simulink model "gm_whdlOFDMTx"  (R2022b)
settings: Solver=FixedStepDiscrete  StartTime=0.0  StopTime=0  RelTol=1e-3
model workspace (MATLAB code in the model file):
  | config = whdlexamples.OFDMTxParameters();
  | fftLen = config.fftLen;
  | subC = config.subC;
  | cpLen = config.cpLen;
  | fs = config.fs;
  | NSS = config.NSS;
  | NRS = config.NRS;
  | NHeader = config.NHeader;
  | NData = config.NData;
  | NSymPerF = config.NSymPerF;
  | ssSymbol = config.ssSymbol;
  | rsSymbol = config.rsSymbol;
  | NHeaderBits = config.NHeaderBits;
  | headerCRCBool = config.headerCRCBool;
  | headerConvK = config.headerConvK;
  | headerConvCode = config.headerConvCode;
  | pilotValPerSym = config.pilotValPerSym;
  | pilotLen = config.pilotLen;
  | dataCRCPoly = config.dataCRCPoly;
  | dataCRCBool = config.dataCRCBool;
  | dataCRCLen = config.dataCRCLen;
  | dataConvK = config.dataConvK;
  | dataConvCode = config.dataConvCode;
  | scramInit = config.scramInit;
  | firCoeff = config.firCoeff;
  | rateFac1 = config.rateFac1;
  | rateFac2 = config.rateFac2;
  | headerLat = config.headerLat;
  | headerTime = config.headerTime;
  | preambleInd = config.preambleInd;
  | headerDataInd = config.headerDataInd;
  | trBlkSize = config.trBlkSize;
  | randOFDM = config.randOFDM;
  | headerIntrlvMaxBlkSize = config.headerIntrlvMaxBlkSize;
  | headerIntrlvNColumns   = config.headerIntrlvNColumns;
  | dataIntrlvMaxBlkSize   = config.dataIntrlvMaxBlkSize;
  | dataIntrlvNColumns     = config.dataIntrlvNColumns;
  | clear config
libraries: hdlsllib x49, simulink x22, dspsigops x11, whdlmod x3, whdledac x3, whdlutilities x2, commhdlcrc x2, dsphdlfiltering2 x1
(part 1 of 4)
settings Model: DataDictionary=whdlOFDMTxData.sldd  Creator=The MathWorks, Inc.  LastModifiedBy=Marwan
settings SolverCC: AlgebraicLoopSolver=TrustRegion  MaxZcPerStep=1
settings DataIOCC: VisualizeSimOutput=off  SaveTime=off  ReturnWorkspaceOutputs=off
settings OptimizationCC: BlockReduction=off  ConditionallyExecuteInputs=off  DefaultParameterBehavior=Inlined  InitFltsAndDblsToZero=on  EfficientMapNaN2IntZero=off
settings DebuggingCC: StringTruncationChecking=none  AlgebraicLoopMsg=error  InheritedTsInSrcMsg=none  SingleTaskRateTransMsg=error  UnconnectedInputMsg=warning  UnconnectedOutputMsg=warning  UnconnectedLineMsg=warning  SFMachineParentedDataDiag=warning
settings HardwareCC: ProdBitPerPointer=32  ProdBitPerSizeT=32  ProdBitPerPtrDiffT=32  ProdLargestAtomicFloat=None  ProdIntDivRoundTo=Undefined  ProdEndianess=Unspecified  ProdWordSize=32  ProdHWDeviceType=ASIC/FPGA->ASIC/FPGA  TargetBitPerPointer=64  TargetBitPerSizeT=64  TargetBitPerPtrDiffT=64  TargetLongLongMode=on  TargetIntDivRoundTo=Zero  TargetEndianess=LittleEndian  TargetWordSize=64  TargetHWDeviceType=Custom Processor->MATLAB Host Computer  ProdEqTarget=off
settings ModelReferenceCC: UpdateModelReferenceTargets=IfOutOfDate  EnableRefExpFcnMdlSchedulingChecks=on  ModelReferenceNumInstancesAllowed=Single
settings RTWCC: RTWVerbose=off  DLArmComputeVersion=19.05
settings CodeAppCC: GenerateComments=off  MaxIdLength=128

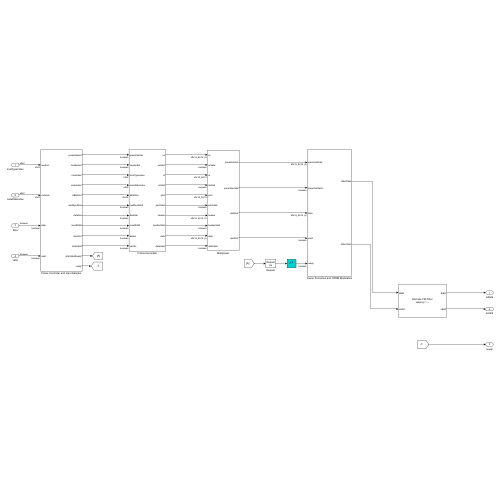
[thumbnail: Simulink's stored preview of the top-level diagram]
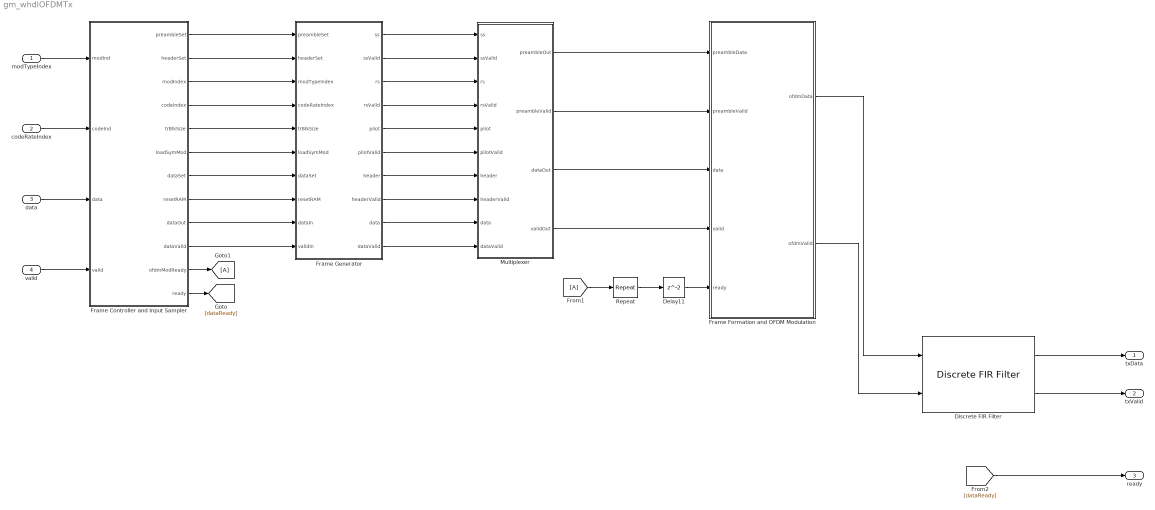
== system gm_whdlOFDMTx ==
  modTypeIndex : Inport  OutDataTypeStr=fixdt(0, 2, 0)  PortDimensions=1  SampleTime=4.8828125e-07
  codeRateIndex : Inport  Port=2  OutDataTypeStr=fixdt(0, 2, 0)  PortDimensions=1  SampleTime=4.8828125e-07
  data : Inport  Port=3  OutDataTypeStr=boolean  PortDimensions=1  SampleTime=4.8828125e-07
  valid : Inport  Port=4  OutDataTypeStr=boolean  PortDimensions=1  SampleTime=4.8828125e-07
  Delay11 : Delay
  Discrete FIR Filter : dsphdlfiltering2/Discrete FIR Filter  NumeratorSource=Property  Numerator=firCoeff  NumeratorPrototype=[]  FilterStructure=Direct form systolic  SerializationOption=Minimum number of cycles between valid input samples  NumCycles=2  NumberOfMultipliers=2  SimulateUsing=Code generation  roundingMode=Floor  overflowMode=off  CoefficientsDataTypeStr=Inherit: Same word length as input  OutputDataTypeStr=Inherit: Same word length as input  ResetInputPort=off  HDLGlobalReset=off
  Frame Controller and Input Sampler : Subsystem
  Frame Formation and OFDM Modulation : Subsystem
  Frame Generator : Subsystem
  From1 : From
  Goto1 : Goto
  Multiplexer : Subsystem
  Repeat : dspsigops/Repeat  N=2  RateOptions=Allow multirate processing  ic=0  mode=Unused parameter value
  txData : Outport  SampleTime=7.8125e-06  VectorParamsAs1DForOutWhenUnconnected=off
  txValid : Outport  Port=2  SampleTime=7.8125e-06  VectorParamsAs1DForOutWhenUnconnected=off
  ready : Outport  Port=3  SampleTime=4.8828125e-07  VectorParamsAs1DForOutWhenUnconnected=off
  wires:
  modTypeIndex/1 -> Frame Controller and Input Sampler/1(modInd)
  codeRateIndex/1 -> Frame Controller and Input Sampler/2(codeInd)
  data/1 -> Frame Controller and Input Sampler/3(data)
  valid/1 -> Frame Controller and Input Sampler/4(valid)
  Delay11/1 -> Frame Formation and OFDM Modulation/5(ready)
  Discrete FIR Filter/1 -> txData/1
  Discrete FIR Filter/2 -> txValid/1
  Frame Controller and Input Sampler/1(preambleSet) -> Frame Generator/1(preambleSet)
  Frame Controller and Input Sampler/2(headerSet) -> Frame Generator/2(headerSet)
  Frame Controller and Input Sampler/3(modIndex) -> Frame Generator/3(modTypeIndex)
  Frame Controller and Input Sampler/4(codeIndex) -> Frame Generator/4(codeRateIndex)
  Frame Controller and Input Sampler/5(trBlkSize) -> Frame Generator/5(trBlkSize)
  Frame Controller and Input Sampler/6(loadSymMod) -> Frame Generator/6(loadSymMod)
  Frame Controller and Input Sampler/7(dataSet) -> Frame Generator/7(dataSet)
  Frame Controller and Input Sampler/8(resetRAM) -> Frame Generator/8(resetRAM)
  Frame Controller and Input Sampler/9(dataOut) -> Frame Generator/9(dataIn)
  Frame Controller and Input Sampler/10(dataValid) -> Frame Generator/10(validIn)
  Frame Controller and Input Sampler/11(ofdmModReady) -> Goto1/1
  Frame Controller and Input Sampler/12(ready) -> [dataReady]
  Frame Formation and OFDM Modulation/1(ofdmData) -> Discrete FIR Filter/1
  Frame Formation and OFDM Modulation/2(ofdmValid) -> Discrete FIR Filter/2
  Frame Generator/1(ss) -> Multiplexer/1(ss)
  Frame Generator/2(ssValid) -> Multiplexer/2(ssValid)
  Frame Generator/3(rs) -> Multiplexer/3(rs)
  Frame Generator/4(rsValid) -> Multiplexer/4(rsValid)
  Frame Generator/5(pilot) -> Multiplexer/5(pilot)
  Frame Generator/6(pilotValid) -> Multiplexer/6(pilotValid)
  Frame Generator/7(header) -> Multiplexer/7(header)
  Frame Generator/8(headerValid) -> Multiplexer/8(headerValid)
  Frame Generator/9(data) -> Multiplexer/9(data)
  Frame Generator/10(dataValid) -> Multiplexer/10(dataValid)
  From1/1 -> Repeat/1
  [dataReady] -> ready/1
  Multiplexer/1(preambleOut) -> Frame Formation and OFDM Modulation/1(preambleData)
  Multiplexer/2(preambleValid) -> Frame Formation and OFDM Modulation/2(preambleValid)
  Multiplexer/3(dataOut) -> Frame Formation and OFDM Modulation/3(data)
  Multiplexer/4(validOut) -> Frame Formation and OFDM Modulation/4(valid)
  Repeat/1 -> Delay11/1

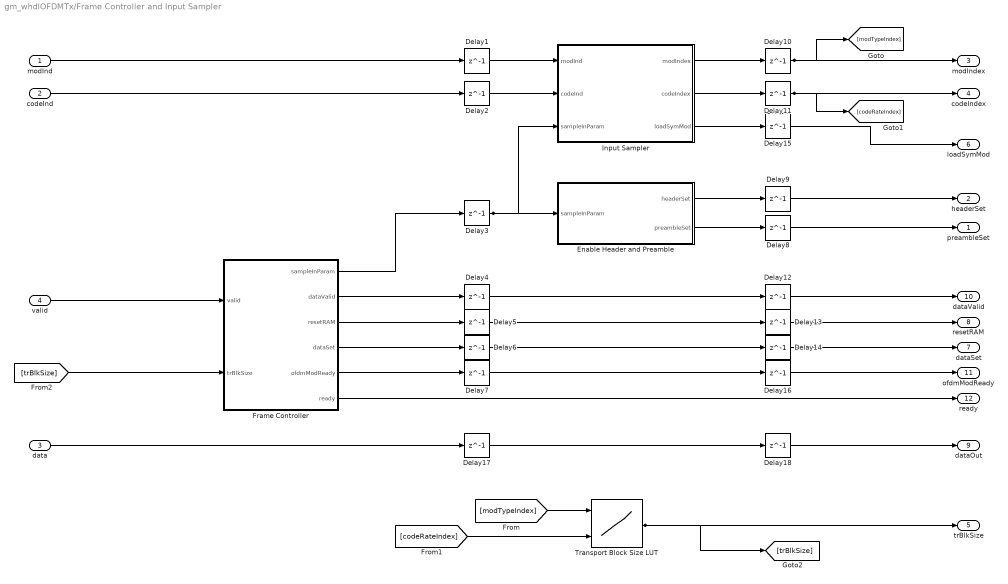
== system gm_whdlOFDMTx/Frame Controller and Input Sampler ==
  modInd : Inport  OutDataTypeStr=fixdt(0, 2, 0)  PortDimensions=1  SampleTime=4.8828125e-07
  codeInd : Inport  Port=2  OutDataTypeStr=fixdt(0, 2, 0)  PortDimensions=1  SampleTime=4.8828125e-07
  data : Inport  Port=3  OutDataTypeStr=boolean  PortDimensions=1  SampleTime=4.8828125e-07
  valid : Inport  Port=4  OutDataTypeStr=boolean  PortDimensions=1  SampleTime=4.8828125e-07
  Delay{1..18} (18 alike) : Delay  DelayLength=1
  "Enable Header and Preamble " : Subsystem
  Frame Controller : Subsystem
  Input Sampler : Subsystem
  Transport Block Size LUT : Lookup_n-D  BreakpointsForDimension1=0:3  BreakpointsForDimension2=0:3  IndexSearchMethod=Evenly spaced points  Table=trBlkSize  ExtrapMethod=Clip  DiagnosticForOutOfRangeInput=Error  UseLastTableValue=on  InternalRulePriority=Speed  OutDataTypeStr=fixdt(0,nextpow2(max(max(trBlkSize)) +1),0)  RndMeth=Simplest
      settings: InputPortMap=u0,u1
  preambleSet : Outport  SampleTime=4.8828125e-07
  headerSet : Outport  Port=2  SampleTime=4.8828125e-07
  modIndex : Outport  Port=3  SampleTime=4.8828125e-07
  codeIndex : Outport  Port=4  SampleTime=4.8828125e-07
  trBlkSize : Outport  Port=5  SampleTime=4.8828125e-07
  loadSymMod : Outport  Port=6  SampleTime=4.8828125e-07
  dataSet : Outport  Port=7  SampleTime=4.8828125e-07
  resetRAM : Outport  Port=8  SampleTime=4.8828125e-07
  dataOut : Outport  Port=9  SampleTime=4.8828125e-07
  dataValid : Outport  Port=10  SampleTime=4.8828125e-07
  ofdmModReady : Outport  Port=11  SampleTime=4.8828125e-07
  ready : Outport  Port=12  SampleTime=4.8828125e-07
  wires:
  modInd/1 -> Delay1/1
  codeInd/1 -> Delay2/1
  data/1 -> Delay17/1
  valid/1 -> Frame Controller/1(valid)
  Delay1/1 -> Input Sampler/1(modInd)
  Delay10/1 -> [modTypeIndex], modIndex/1
  Delay11/1 -> [codeRateIndex], codeIndex/1
  Delay12/1 -> dataValid/1
  Delay13/1 -> resetRAM/1
  Delay14/1 -> dataSet/1
  Delay15/1 -> loadSymMod/1
  Delay16/1 -> ofdmModReady/1
  Delay17/1 -> Delay18/1
  Delay18/1 -> dataOut/1
  Delay2/1 -> Input Sampler/2(codeInd)
  Delay3/1 -> Input Sampler/3(sampleInParam), "Enable Header and Preamble "/1(sampleInParam)
  Delay4/1 -> Delay12/1
  Delay5/1 -> Delay13/1
  Delay6/1 -> Delay14/1
  Delay7/1 -> Delay16/1
  Delay8/1 -> preambleSet/1
  Delay9/1 -> headerSet/1
  "Enable Header and Preamble "/1(headerSet) -> Delay9/1
  "Enable Header and Preamble "/2(preambleSet) -> Delay8/1
  Frame Controller/1(sampleInParam) -> Delay3/1
  Frame Controller/2(dataValid) -> Delay4/1
  Frame Controller/3(resetRAM) -> Delay5/1
  Frame Controller/4(dataSet) -> Delay6/1
  Frame Controller/5(ofdmModReady) -> Delay7/1
  Frame Controller/6(ready) -> ready/1
  [modTypeIndex] -> Transport Block Size LUT/1
  [codeRateIndex] -> Transport Block Size LUT/2
  [trBlkSize] -> Frame Controller/2(trBlkSize)
  Input Sampler/1(modIndex) -> Delay10/1
  Input Sampler/2(codeIndex) -> Delay11/1
  Input Sampler/3(loadSymMod) -> Delay15/1
  Transport Block Size LUT/1 -> [trBlkSize], trBlkSize/1

== system gm_whdlOFDMTx/Frame Formation and OFDM Modulation ==
  preambleData : Inport  OutDataTypeStr=fixdt(1, 16, 14)  PortDimensions=1  SampleTime=2.44140625e-07
      settings: SignalType=complex
  preambleValid : Inport  Port=2  OutDataTypeStr=boolean  PortDimensions=1  SampleTime=2.44140625e-07
  data : Inport  Port=3  OutDataTypeStr=fixdt(1, 16, 14)  PortDimensions=1  SampleTime=2.44140625e-07
      settings: SignalType=complex
  valid : Inport  Port=4  OutDataTypeStr=boolean  PortDimensions=1  SampleTime=2.44140625e-07
  ready : Inport  Port=5  OutDataTypeStr=boolean  PortDimensions=1  SampleTime=2.44140625e-07
  Complex to Real-Imag : ComplexToRealImag  Output=Real
  Data Type Conversion : DataTypeConversion  SaturateOnIntegerOverflow=off  RndMeth=Floor
  Delay3 : Delay  DelayLength=1
  Downsample : DownSample  N=rateFac1  RateOptions=Allow multirate processing
  Dual Rate RAM : hdlsllib/HDL RAMs/Dual Rate Dual Port RAM  ram_size=nextpow2(subC*NSymPerF +1)
  Dual Rate RAM_term0 : Terminator
  Generate OFDM Modulator Valid : Subsystem
  Generate RAM Inputs : Subsystem
  Make OFDM Valid Continuous : Subsystem
  OFDM Modulator : Subsystem
  constant : Constant  Value=complex(0)  OutDataTypeStr=Inherit: Inherit via back propagation  SampleTime=-1
  ofdmData : Outport  SampleTime=7.8125e-06  VectorParamsAs1DForOutWhenUnconnected=off
  ofdmValid : Outport  Port=2  SampleTime=7.8125e-06  VectorParamsAs1DForOutWhenUnconnected=off
  wires:
  preambleData/1 -> Generate RAM Inputs/1(preambleData)
  preambleValid/1 -> Generate RAM Inputs/2(enb)
  data/1 -> Generate RAM Inputs/3(data)
  valid/1 -> Generate RAM Inputs/4(valid)
  ready/1 -> Downsample/1
  Complex to Real-Imag/1 -> Data Type Conversion/1
  Data Type Conversion/1 -> Dual Rate RAM/6
  Delay3/1 -> Generate OFDM Modulator Valid/2(ofdmModReady)
  Downsample/1 -> Generate OFDM Modulator Valid/1(generatedReady)
  Dual Rate RAM/1 -> Dual Rate RAM_term0/1
  Dual Rate RAM/2 -> OFDM Modulator/1(data)
  Generate OFDM Modulator Valid/1(RAMAddress) -> Dual Rate RAM/5
  Generate OFDM Modulator Valid/2(ofdmModValid) -> OFDM Modulator/2(valid)
  Generate RAM Inputs/1(RAMData) -> Dual Rate RAM/1
  Generate RAM Inputs/2(RAMAddress) -> Dual Rate RAM/2
  Generate RAM Inputs/3(RAMValid) -> Dual Rate RAM/3
  Make OFDM Valid Continuous/1(ofdmData) -> ofdmData/1
  Make OFDM Valid Continuous/2(ofdmValid) -> ofdmValid/1
  OFDM Modulator/1(data1) -> Make OFDM Valid Continuous/1(dataIn)
  OFDM Modulator/2(valid1) -> Make OFDM Valid Continuous/2(validIn)
  OFDM Modulator/3(ready) -> Delay3/1
  constant/1 -> Complex to Real-Imag/1, Dual Rate RAM/4

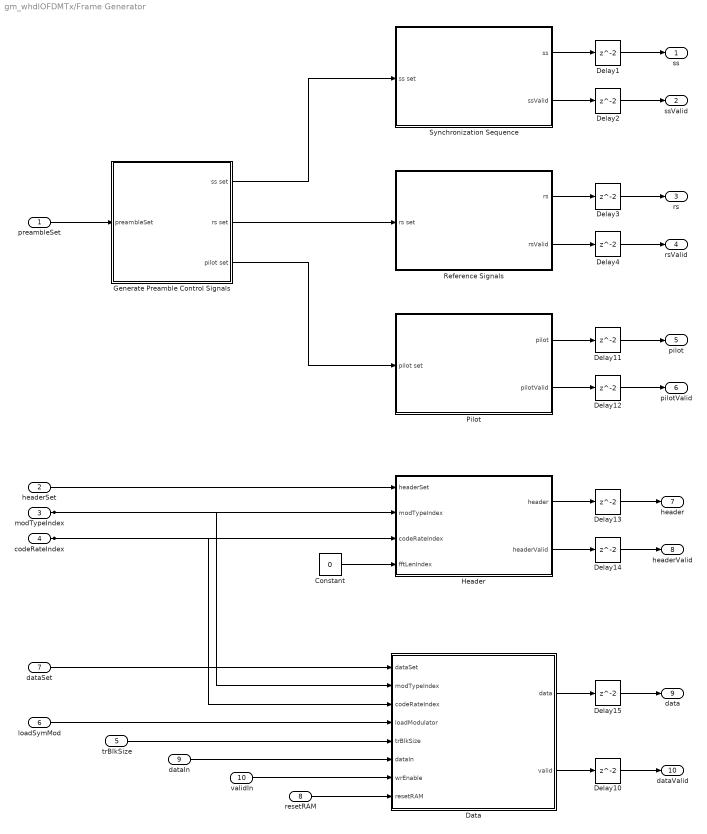
== system gm_whdlOFDMTx/Frame Generator ==
  preambleSet : Inport  OutDataTypeStr=boolean  PortDimensions=1  SampleTime=4.8828125e-07
  headerSet : Inport  Port=2  OutDataTypeStr=boolean  PortDimensions=1  SampleTime=4.8828125e-07
  modTypeIndex : Inport  Port=3  OutDataTypeStr=fixdt(0, 2, 0)  PortDimensions=1  SampleTime=4.8828125e-07
  codeRateIndex : Inport  Port=4  OutDataTypeStr=fixdt(0, 2, 0)  PortDimensions=1  SampleTime=4.8828125e-07
  trBlkSize : Inport  Port=5  OutDataTypeStr=fixdt(0, 14, 0)  PortDimensions=1  SampleTime=4.8828125e-07
  loadSymMod : Inport  Port=6  OutDataTypeStr=boolean  PortDimensions=1  SampleTime=4.8828125e-07
  dataSet : Inport  Port=7  OutDataTypeStr=boolean  PortDimensions=1  SampleTime=4.8828125e-07
  resetRAM : Inport  Port=8  OutDataTypeStr=boolean  PortDimensions=1  SampleTime=4.8828125e-07
  dataIn : Inport  Port=9  OutDataTypeStr=boolean  PortDimensions=1  SampleTime=4.8828125e-07
  validIn : Inport  Port=10  OutDataTypeStr=boolean  PortDimensions=1  SampleTime=4.8828125e-07
  Constant : Constant  Value=0  OutDataTypeStr=fixdt(0,3,0)  SampleTime=-1
  Data : Subsystem
  Delay{1..4,10..15} (10 alike) : Delay
  Generate Preamble Control Signals : Subsystem
  Header : Subsystem
  Pilot : Subsystem
  Reference Signals : Subsystem
  Synchronization Sequence : Subsystem
  ss : Outport  SampleTime=2.44140625e-07
  ssValid : Outport  Port=2  SampleTime=2.44140625e-07
  rs : Outport  Port=3  SampleTime=2.44140625e-07
  rsValid : Outport  Port=4  SampleTime=2.44140625e-07
  pilot : Outport  Port=5  SampleTime=2.44140625e-07
  pilotValid : Outport  Port=6  SampleTime=2.44140625e-07
  header : Outport  Port=7  SampleTime=2.44140625e-07
  headerValid : Outport  Port=8  SampleTime=2.44140625e-07
  data : Outport  Port=9  SampleTime=2.44140625e-07
  dataValid : Outport  Port=10  SampleTime=2.44140625e-07
  wires:
  preambleSet/1 -> Generate Preamble Control Signals/1(preambleSet)
  headerSet/1 -> Header/1(headerSet)
  modTypeIndex/1 -> Data/2(modTypeIndex), Header/2(modTypeIndex)
  codeRateIndex/1 -> Data/3(codeRateIndex), Header/3(codeRateIndex)
  trBlkSize/1 -> Data/5(trBlkSize)
  loadSymMod/1 -> Data/4(loadModulator)
  dataSet/1 -> Data/1(dataSet)
  resetRAM/1 -> Data/8(resetRAM)
  dataIn/1 -> Data/6(dataIn)
  validIn/1 -> Data/7(wrEnable)
  Constant/1 -> Header/4(fftLenIndex)
  Data/1(data) -> Delay15/1
  Data/2(valid) -> Delay10/1
  Delay1/1 -> ss/1
  Delay10/1 -> dataValid/1
  Delay11/1 -> pilot/1
  Delay12/1 -> pilotValid/1
  Delay13/1 -> header/1
  Delay14/1 -> headerValid/1
  Delay15/1 -> data/1
  Delay2/1 -> ssValid/1
  Delay3/1 -> rs/1
  Delay4/1 -> rsValid/1
  Generate Preamble Control Signals/1(ss set) -> Synchronization Sequence/1(ss set)
  Generate Preamble Control Signals/2(rs set) -> Reference Signals/1(rs set)
  Generate Preamble Control Signals/3(pilot set) -> Pilot/1(pilot set)
  Header/1(header) -> Delay13/1
  Header/2(headerValid) -> Delay14/1
  Pilot/1(pilot) -> Delay11/1
  Pilot/2(pilotValid) -> Delay12/1
  Reference Signals/1(rs) -> Delay3/1
  Reference Signals/2(rsValid) -> Delay4/1
  Synchronization Sequence/1(ss) -> Delay1/1
  Synchronization Sequence/2(ssValid) -> Delay2/1

== system gm_whdlOFDMTx/Multiplexer ==
  ss : Inport  OutDataTypeStr=fixdt(1, 16, 14)  PortDimensions=1  SampleTime=2.44140625e-07
      settings: SignalType=complex
  ssValid : Inport  Port=2  OutDataTypeStr=boolean  PortDimensions=1  SampleTime=2.44140625e-07
  rs : Inport  Port=3  OutDataTypeStr=fixdt(1, 16, 14)  PortDimensions=1  SampleTime=2.44140625e-07
  rsValid : Inport  Port=4  OutDataTypeStr=boolean  PortDimensions=1  SampleTime=2.44140625e-07
  pilot : Inport  Port=5  OutDataTypeStr=fixdt(1, 16, 14)  PortDimensions=1  SampleTime=2.44140625e-07
  pilotValid : Inport  Port=6  OutDataTypeStr=boolean  PortDimensions=1  SampleTime=2.44140625e-07
  header : Inport  Port=7  OutDataTypeStr=fixdt(1, 16, 14)  PortDimensions=1  SampleTime=2.44140625e-07
      settings: SignalType=complex
  headerValid : Inport  Port=8  OutDataTypeStr=boolean  PortDimensions=1  SampleTime=2.44140625e-07
  data : Inport  Port=9  OutDataTypeStr=fixdt(1, 16, 14)  PortDimensions=1  SampleTime=2.44140625e-07
      settings: SignalType=complex
  dataValid : Inport  Port=10  OutDataTypeStr=boolean  PortDimensions=1  SampleTime=2.44140625e-07
  Multiplex Header and Data Signals : Subsystem
  Multiplex Preamble Signals : Subsystem
  preambleOut : Outport  SampleTime=2.44140625e-07
  preambleValid : Outport  Port=2  SampleTime=2.44140625e-07
  dataOut : Outport  Port=3  SampleTime=2.44140625e-07
  validOut : Outport  Port=4  SampleTime=2.44140625e-07
  wires:
  ss/1 -> Multiplex Preamble Signals/1(ss)
  ssValid/1 -> Multiplex Preamble Signals/2(ssValid)
  rs/1 -> Multiplex Preamble Signals/3(rs)
  rsValid/1 -> Multiplex Preamble Signals/4(rsValid)
  pilot/1 -> Multiplex Preamble Signals/5(pilot)
  pilotValid/1 -> Multiplex Preamble Signals/6(pilotValid)
  header/1 -> Multiplex Header and Data Signals/1(header)
  headerValid/1 -> Multiplex Header and Data Signals/2(headerValid)
  data/1 -> Multiplex Header and Data Signals/3(data)
  dataValid/1 -> Multiplex Header and Data Signals/4(dataValid)
  Multiplex Header and Data Signals/1(dataOut) -> dataOut/1
  Multiplex Header and Data Signals/2(validOut) -> validOut/1
  Multiplex Preamble Signals/1(preambleOut) -> preambleOut/1
  Multiplex Preamble Signals/2(preambleValid) -> preambleValid/1

== system gm_whdlOFDMTx/Frame Controller and Input Sampler/Enable Header and Preamble  ==
  sampleInParam : Inport  OutDataTypeStr=boolean  PortDimensions=1  SampleTime=4.8828125e-07
  Constant1 : Constant  Value=false  SampleTime=-1
  Delay2 : Delay  DelayLength=1
  Falling Edge Detector1 : Subsystem
  Falling Edge Detector2 : Subsystem
  MATLAB Function3 : Subsystem
  MATLAB Function4 : Subsystem
  Unit Delay Enabled Synchronous : hdlsllib/Discrete/Unit Delay Enabled Synchronous  InitialCondition=1  SampleTime=-1
  headerSet : Outport  SampleTime=4.8828125e-07
  preambleSet : Outport  Port=2  SampleTime=4.8828125e-07
  wires:
  sampleInParam/1 -> Delay2/1, MATLAB Function3/1(trigger)
  Constant1/1 -> Unit Delay Enabled Synchronous/1
  Delay2/1 -> headerSet/1
  Falling Edge Detector1/1(out) -> Unit Delay Enabled Synchronous/2
  Falling Edge Detector2/1(out) -> MATLAB Function4/1(trigger)
  MATLAB Function3/1(out) -> Falling Edge Detector1/1(in)
  MATLAB Function4/1(out) -> preambleSet/1
  Unit Delay Enabled Synchronous/1 -> Falling Edge Detector2/1(in)

== system gm_whdlOFDMTx/Frame Controller and Input Sampler/Frame Controller ==
  valid : Inport  OutDataTypeStr=boolean  PortDimensions=1  SampleTime=4.8828125e-07
  trBlkSize : Inport  Port=2  OutDataTypeStr=fixdt(0, 14, 0)  PortDimensions=1  SampleTime=4.8828125e-07
  Delay : Delay  DelayLength=1
  Generate OFDM Modulator Ready : Subsystem
  Generate Transmitter Ready : Subsystem
  sampleInParam : Outport  SampleTime=4.8828125e-07
  dataValid : Outport  Port=2  SampleTime=4.8828125e-07
  resetRAM : Outport  Port=3  SampleTime=4.8828125e-07
  dataSet : Outport  Port=4  SampleTime=4.8828125e-07
  ofdmModReady : Outport  Port=5  SampleTime=4.8828125e-07
  ready : Outport  Port=6  SampleTime=4.8828125e-07
  wires:
  valid/1 -> Generate Transmitter Ready/1(valid)
  trBlkSize/1 -> Generate OFDM Modulator Ready/2(trBlkSize), Generate Transmitter Ready/3(trBlkSize)
  Delay/1 -> Generate Transmitter Ready/2(reset)
  Generate OFDM Modulator Ready/1(resetRAM) -> resetRAM/1
  Generate OFDM Modulator Ready/2(dataSet) -> dataSet/1
  Generate OFDM Modulator Ready/3(ofdmModReady) -> ofdmModReady/1
  Generate OFDM Modulator Ready/4(reset) -> Delay/1
  Generate Transmitter Ready/1(sampleInParam) -> sampleInParam/1
  Generate Transmitter Ready/2(dataValid) -> dataValid/1
  Generate Transmitter Ready/3(ready) -> Generate OFDM Modulator Ready/1(ready), ready/1

== system gm_whdlOFDMTx/Frame Controller and Input Sampler/Input Sampler ==
  modInd : Inport  OutDataTypeStr=fixdt(0, 2, 0)  PortDimensions=1  SampleTime=4.8828125e-07
  codeInd : Inport  Port=2  OutDataTypeStr=fixdt(0, 2, 0)  PortDimensions=1  SampleTime=4.8828125e-07
  sampleInParam : Inport  Port=3  OutDataTypeStr=boolean  PortDimensions=1  SampleTime=4.8828125e-07
  Delay : Delay  DelayLength=1
  Unit Delay Enabled Synchronous : hdlsllib/Discrete/Unit Delay Enabled Synchronous  InitialCondition=1  SampleTime=-1
  Unit Delay Enabled Synchronous1 : hdlsllib/Discrete/Unit Delay Enabled Synchronous  InitialCondition=0  SampleTime=-1
  modIndex : Outport  SampleTime=4.8828125e-07
  codeIndex : Outport  Port=2  SampleTime=4.8828125e-07
  loadSymMod : Outport  Port=3  SampleTime=4.8828125e-07
  wires:
  modInd/1 -> Unit Delay Enabled Synchronous/1
  codeInd/1 -> Unit Delay Enabled Synchronous1/1
  sampleInParam/1 -> Unit Delay Enabled Synchronous1/2, Unit Delay Enabled Synchronous/2, Delay/1
  Delay/1 -> loadSymMod/1
  Unit Delay Enabled Synchronous/1 -> modIndex/1
  Unit Delay Enabled Synchronous1/1 -> codeIndex/1

== system gm_whdlOFDMTx/Frame Formation and OFDM Modulation/Generate OFDM Modulator Valid ==
  generatedReady : Inport  OutDataTypeStr=boolean  PortDimensions=1  SampleTime=7.8125e-06
  ofdmModReady : Inport  Port=2  OutDataTypeStr=boolean  PortDimensions=1  SampleTime=7.8125e-06
  Constant : Constant  Value=subC*NSymPerF  OutDataTypeStr=Inherit: Inherit via back propagation  SampleTime=-1
  Counter for Read Address : Subsystem
  Delay : Delay
  Logical Operator4 : Logic  IconShape=distinctive  AllPortsSameDT=off  OutDataTypeStr=boolean
  Switch : Switch  Criteria=u2 ~= 0  OutDataTypeStr=Inherit: Inherit via back propagation  SaturateOnIntegerOverflow=off  InputSameDT=off
  RAMAddress : Outport  SampleTime=7.8125e-06
  ofdmModValid : Outport  Port=2  SampleTime=7.8125e-06
  wires:
  generatedReady/1 -> Switch/2, Delay/1
  ofdmModReady/1 -> Logical Operator4/2
  Constant/1 -> Switch/3
  Counter for Read Address/1(out) -> Switch/1
  Delay/1 -> Logical Operator4/1
  Logical Operator4/1 -> Counter for Read Address/1(enableIn), ofdmModValid/1
  Switch/1 -> RAMAddress/1

== system gm_whdlOFDMTx/Frame Formation and OFDM Modulation/Generate RAM Inputs ==
  preambleData : Inport  OutDataTypeStr=fixdt(1, 16, 14)  PortDimensions=1  SampleTime=2.44140625e-07
      settings: SignalType=complex
  enb : Inport  Port=2  OutDataTypeStr=boolean  PortDimensions=1  SampleTime=2.44140625e-07
  data : Inport  Port=3  OutDataTypeStr=fixdt(1, 16, 14)  PortDimensions=1  SampleTime=2.44140625e-07
      settings: SignalType=complex
  valid : Inport  Port=4  OutDataTypeStr=boolean  PortDimensions=1  SampleTime=2.44140625e-07
  Delay{,1..4} (5 alike) : Delay  DelayLength=1
  HDL Counter : hdlsllib/Sources/HDL Counter  CountType=Count limited  CountInit=0  CountStep=1  CountMax=length(preambleInd) -1  CountFromType=Initial value  CountFrom=0  CountResetPort=off  CountLoadPort=off  CountEnbPort=on  CountDirPort=off  CountHitOutputPort=off  CountDataType=Unsigned  CountWordLen=nextpow2(length(preambleInd))  CountFracLen=0  CountSampTime=1
  HDL Counter1 : hdlsllib/Sources/HDL Counter  CountType=Count limited  CountInit=0  CountStep=1  CountMax=length(headerDataInd) -1  CountFromType=Initial value  CountFrom=0  CountResetPort=off  CountLoadPort=off  CountEnbPort=on  CountDirPort=off  CountHitOutputPort=off  CountDataType=Unsigned  CountWordLen=nextpow2(length(headerDataInd))  CountFracLen=0  CountSampTime=1
  Header Data Indices LUT : Lookup_n-D  NumberOfTableDimensions=1  LookupTableObject=''  BreakpointsForDimension1=0:(length(headerDataInd) -1)  BreakpointsForDimension1FirstPoint=10  BreakpointsForDimension2FirstPoint=10  BreakpointsForDimension1Spacing=12  BreakpointsForDimension2Spacing=12  IndexSearchMethod=Evenly spaced points  Table=headerDataInd - 1  TableDataTypeStr=fixdt(0,nextpow2((NSymPerF*subC) +1),0)  InterpMethod=Flat  DiagnosticForOutOfRangeInput=Error  InternalRulePriority=Speed  OutDataTypeStr=fixdt(0,nextpow2((NSymPerF*subC) +1),0)  RndMeth=Simplest
  Logical Operator : Logic  Operator=OR  IconShape=distinctive  AllPortsSameDT=off  OutDataTypeStr=boolean
  Preamble Indices LUT : Lookup_n-D  NumberOfTableDimensions=1  LookupTableObject=''  BreakpointsForDimension1=0:(length(preambleInd) -1)  BreakpointsForDimension1FirstPoint=10  BreakpointsForDimension2FirstPoint=10  BreakpointsForDimension1Spacing=12  BreakpointsForDimension2Spacing=12  IndexSearchMethod=Evenly spaced points  Table=preambleInd - 1  TableDataTypeStr=fixdt(0,nextpow2((NSymPerF*subC) +1),0)  InterpMethod=Flat  DiagnosticForOutOfRangeInput=Error  InternalRulePriority=Speed  OutDataTypeStr=fixdt(0,nextpow2((NSymPerF*subC) +1),0)  RndMeth=Simplest
  Switch : Switch  Criteria=u2 ~= 0  SaturateOnIntegerOverflow=off  InputSameDT=off
  Switch1 : Switch  Criteria=u2 ~= 0  SaturateOnIntegerOverflow=off  InputSameDT=off
  RAMData : Outport  SampleTime=2.44140625e-07
  RAMAddress : Outport  Port=2  SampleTime=2.44140625e-07
  RAMValid : Outport  Port=3  SampleTime=2.44140625e-07
  wires:
  preambleData/1 -> Switch1/1
  enb/1 -> Switch1/2, Logical Operator/1, Delay1/1, HDL Counter/1
  data/1 -> Switch1/3
  valid/1 -> Logical Operator/2, HDL Counter1/1
  Delay/1 -> Switch/1
  Delay1/1 -> Switch/2
  Delay2/1 -> Switch/3
  Delay3/1 -> RAMData/1
  Delay4/1 -> RAMValid/1
  HDL Counter/1 -> Preamble Indices LUT/1
  HDL Counter1/1 -> Header Data Indices LUT/1
  Header Data Indices LUT/1 -> Delay2/1
  Logical Operator/1 -> Delay4/1
  Preamble Indices LUT/1 -> Delay/1
  Switch/1 -> RAMAddress/1
  Switch1/1 -> Delay3/1

== system gm_whdlOFDMTx/Frame Formation and OFDM Modulation/Make OFDM Valid Continuous ==
  dataIn : Inport  OutDataTypeStr=fixdt(1, 16, 14)  PortDimensions=1  SampleTime=7.8125e-06
      settings: SignalType=complex
  validIn : Inport  Port=2  OutDataTypeStr=boolean  PortDimensions=1  SampleTime=7.8125e-06
  Constant : Constant  Value=complex(0)  OutDataTypeStr=Inherit: Inherit via back propagation  SampleTime=-1
  Delay{,1..3} (4 alike) : Delay  DelayLength=1
  Random OFDM Symbol : Subsystem
  Rising Edge Detector : Subsystem
  Switch : Switch  Criteria=u2 ~= 0  SaturateOnIntegerOverflow=off
  Switch1 : Switch  Criteria=u2 ~= 0  SaturateOnIntegerOverflow=off
  Unit Delay Enabled Synchronous : hdlsllib/Discrete/Unit Delay Enabled Synchronous  InitialCondition=0.0  SampleTime=-1
  ofdmData : Outport  SampleTime=7.8125e-06
  ofdmValid : Outport  Port=2  SampleTime=7.8125e-06
  wires:
  dataIn/1 -> Delay2/1
  validIn/1 -> Delay/1, Rising Edge Detector/1(in), Random OFDM Symbol/1(in)
  Constant/1 -> Switch/3
  Delay/1 -> Switch1/2
  Delay1/1 -> Switch/1
  Delay2/1 -> Switch1/1
  Delay3/1 -> Unit Delay Enabled Synchronous/2, Unit Delay Enabled Synchronous/1
  Random OFDM Symbol/1(out) -> Switch1/3
  Rising Edge Detector/1(out) -> Delay3/1
  Switch/1 -> ofdmData/1
  Switch1/1 -> Delay1/1
  Unit Delay Enabled Synchronous/1 -> Switch/2, ofdmValid/1

== system gm_whdlOFDMTx/Frame Formation and OFDM Modulation/OFDM Modulator ==
  data : Inport  OutDataTypeStr=fixdt(1, 16, 14)  SampleTime=7.8125e-06
      settings: SignalType=complex
  valid : Inport  Port=2  OutDataTypeStr=boolean  SampleTime=7.8125e-06
  OFDM Modulator : whdlmod/OFDM Modulator  OFDMParametersSource=Property  FFTLength=fftLen  MaxFFTLength=1024  CPLength=cpLen  numLgSc=(fftLen-subC)/2  numRgSc=(fftLen-subC)/2 -1  InsertDCNull=on  Windowing=off  WindowLength=4  MaxWindowLength=8  ResetInputPort=off  Normalize=on  RoundingMethod=Floor  SimulateUsing=Code generation
  data1 : Outport  SampleTime=7.8125e-06
  valid1 : Outport  Port=2  SampleTime=7.8125e-06
  ready : Outport  Port=3  SampleTime=7.8125e-06
  wires:
  data/1 -> OFDM Modulator/1
  valid/1 -> OFDM Modulator/2
  OFDM Modulator/1 -> data1/1
  OFDM Modulator/2 -> valid1/1
  OFDM Modulator/3 -> ready/1

== system gm_whdlOFDMTx/Frame Generator/Data ==
  dataSet : Inport  OutDataTypeStr=boolean  PortDimensions=1  SampleTime=4.8828125e-07
  modTypeIndex : Inport  Port=2  OutDataTypeStr=fixdt(0, 2, 0)  PortDimensions=1  SampleTime=4.8828125e-07
  codeRateIndex : Inport  Port=3  OutDataTypeStr=fixdt(0, 2, 0)  PortDimensions=1  SampleTime=4.8828125e-07
  loadModulator : Inport  Port=4  OutDataTypeStr=boolean  PortDimensions=1  SampleTime=4.8828125e-07
  trBlkSize : Inport  Port=5  OutDataTypeStr=fixdt(0, 14, 0)  PortDimensions=1  SampleTime=4.8828125e-07
  dataIn : Inport  Port=6  OutDataTypeStr=boolean  PortDimensions=1  SampleTime=4.8828125e-07
  wrEnable : Inport  Port=7  OutDataTypeStr=boolean  PortDimensions=1  SampleTime=4.8828125e-07
  resetRAM : Inport  Port=8  OutDataTypeStr=boolean  PortDimensions=1  SampleTime=4.8828125e-07
  Data Chain : Subsystem
  Data and Control Signal Generation : Subsystem
  data : Outport  SampleTime=2.44140625e-07
  valid : Outport  Port=2  SampleTime=2.44140625e-07
  wires:
  dataSet/1 -> Data and Control Signal Generation/1(dataSet)
  modTypeIndex/1 -> Data and Control Signal Generation/2(modTypeIndex)
  codeRateIndex/1 -> Data and Control Signal Generation/3(codeRateIndex)
  loadModulator/1 -> Data and Control Signal Generation/4(loadMod)
  trBlkSize/1 -> Data and Control Signal Generation/5(trBlkSize)
  dataIn/1 -> Data and Control Signal Generation/6(dataIn)
  wrEnable/1 -> Data and Control Signal Generation/7(wrEnable)
  resetRAM/1 -> Data and Control Signal Generation/8(resetRAM)
  Data Chain/1(data) -> data/1
  Data Chain/2(valid) -> valid/1
  Data and Control Signal Generation/1(data) -> Data Chain/1(dataIn)
  Data and Control Signal Generation/2(start) -> Data Chain/2(startIn)
  Data and Control Signal Generation/3(end) -> Data Chain/3(endIn)
  Data and Control Signal Generation/4(valid) -> Data Chain/4(validIn)
  Data and Control Signal Generation/5(puncVector) -> Data Chain/5(puncVector)
  Data and Control Signal Generation/6(modTypeInd) -> Data Chain/6(modTypeInd)
  Data and Control Signal Generation/7(loadModulator) -> Data Chain/7(loadModulator)

== system gm_whdlOFDMTx/Frame Generator/Generate Preamble Control Signals ==
  preambleSet : Inport  OutDataTypeStr=boolean  PortDimensions=1  SampleTime=4.8828125e-07
  Compare To Constant : simulink/Logic and Bit Operations/Compare To Constant  relop=<  const=NSS*subC  OutDataTypeStr=boolean
  Compare To Constant1 : simulink/Logic and Bit Operations/Compare To Constant  relop=>=  const=NSS*subC  OutDataTypeStr=boolean
  Compare To Constant2 : simulink/Logic and Bit Operations/Compare To Constant  relop=<  const=NSS*subC + NRS*subC  OutDataTypeStr=boolean
  Compare To Constant3 : simulink/Logic and Bit Operations/Compare To Constant  relop=>=  const=NSS*subC + NRS*subC  OutDataTypeStr=boolean
  Compare To Constant4 : simulink/Logic and Bit Operations/Compare To Constant  relop=<  const=NSS*subC + NRS*subC + pilotLen  OutDataTypeStr=boolean
  HDL Counter : hdlsllib/Sources/HDL Counter  CountType=Count limited  CountInit=0  CountStep=1  CountMax=NSS*subC + NRS*subC + pilotLen  CountFromType=Initial value  CountFrom=0  CountResetPort=off  CountLoadPort=off  CountEnbPort=on  CountDirPort=off  CountHitOutputPort=off  CountDataType=Unsigned  CountWordLen=nextpow2(NSS*subC + NRS*subC + pilotLen +1)  CountFracLen=0  CountSampTime=1
  Logical Operator{,1..4} (5 alike) : Logic  IconShape=distinctive  AllPortsSameDT=off  OutDataTypeStr=boolean
  ss set : Outport  SampleTime=4.8828125e-07
  rs set : Outport  Port=2  SampleTime=4.8828125e-07
  pilot set : Outport  Port=3  SampleTime=4.8828125e-07
  wires:
  preambleSet/1 -> Logical Operator4/2, Logical Operator3/2, Logical Operator2/2, HDL Counter/1
  Compare To Constant/1 -> Logical Operator2/1
  Compare To Constant1/1 -> Logical Operator/1
  Compare To Constant2/1 -> Logical Operator/2
  Compare To Constant3/1 -> Logical Operator1/1
  Compare To Constant4/1 -> Logical Operator1/2
  HDL Counter/1 -> Compare To Constant4/1, Compare To Constant3/1, Compare To Constant2/1, Compare To Constant1/1, Compare To Constant/1
  Logical Operator/1 -> Logical Operator3/1
  Logical Operator1/1 -> Logical Operator4/1
  Logical Operator2/1 -> ss set/1
  Logical Operator3/1 -> rs set/1
  Logical Operator4/1 -> pilot set/1

== system gm_whdlOFDMTx/Frame Generator/Header ==
  headerSet : Inport  OutDataTypeStr=boolean  PortDimensions=1  SampleTime=4.8828125e-07
  modTypeIndex : Inport  Port=2  OutDataTypeStr=fixdt(0, 2, 0)  PortDimensions=1  SampleTime=4.8828125e-07
  codeRateIndex : Inport  Port=3  OutDataTypeStr=fixdt(0, 2, 0)  PortDimensions=1  SampleTime=4.8828125e-07
  fftLenIndex : Inport  Port=4  OutDataTypeStr=fixdt(0, 3, 0)  PortDimensions=1  SampleTime=4.8828125e-07
  Convolutional Encoder : whdledac/Convolutional Encoder  ConstraintLength=headerConvK  CodeGenerator=headerConvCode  FeedbackConnection=0  TerminationMethod=Terminated  ResetPort=off  InitialStatePort=off  FinalStatePort=off  SimulateUsing=Code generation
  Create Control Bus : Subsystem
  General CRC Generator HDL Optimized : commhdlcrc/General CRC Generator HDL Optimized  Polynomial=headerCRCBool  InitialState=0  DirectMethod=off  ReflectInput=off  ReflectCRCChecksum=off  FinalXORValue=0  SimulateUsing=Code generation
  Header Formation : Subsystem
  Interleaver : Subsystem  mask{maxBlkSize=double(72), nColumns=double(18)}
      mask prompts: maxBlkSize "Maximum block size:"; nColumns "Number of columns:"
      mask init:
      | maxBlkSize = double(72);
      | maxNRows = double(4);
      | nColumns = double(18);
  Interleaver_term1 : Terminator
  Interleaver_term2 : Terminator
  Interleaver_term4 : Terminator
  LTE Symbol Modulator : Subsystem
  Serializer : Subsystem
  header : Outport  SampleTime=2.44140625e-07
  headerValid : Outport  Port=2  SampleTime=2.44140625e-07
  wires:
  headerSet/1 -> Header Formation/4(validIn)
  modTypeIndex/1 -> Header Formation/1(modType)
  codeRateIndex/1 -> Header Formation/2(codeRate)
  fftLenIndex/1 -> Header Formation/3(fftLen)
  Convolutional Encoder/1 -> Serializer/1(parallelIn)
  Convolutional Encoder/2 -> Serializer/2(ctrlIn)
  Create Control Bus/1(dataOut) -> Convolutional Encoder/1
  Create Control Bus/2(ctrlOut) -> Convolutional Encoder/2
  General CRC Generator HDL Optimized/1 -> Create Control Bus/1(dataIn)
  General CRC Generator HDL Optimized/2 -> Create Control Bus/2(startIn)
  General CRC Generator HDL Optimized/3 -> Create Control Bus/3(endIn)
  General CRC Generator HDL Optimized/4 -> Create Control Bus/4(validIn)
  Header Formation/1(headerBits) -> General CRC Generator HDL Optimized/1
  Header Formation/2(startOut) -> General CRC Generator HDL Optimized/2
  Header Formation/3(endOut) -> General CRC Generator HDL Optimized/3
  Header Formation/4(validOut) -> General CRC Generator HDL Optimized/4
  Interleaver/1(dataOut) -> LTE Symbol Modulator/1(data)
  Interleaver/2(startOut) -> Interleaver_term1/1
  Interleaver/3(endOut) -> Interleaver_term2/1
  Interleaver/4(validOut) -> LTE Symbol Modulator/2(valid)
  Interleaver/5(ready) -> Interleaver_term4/1
  LTE Symbol Modulator/1(data1) -> header/1
  LTE Symbol Modulator/2(valid1) -> headerValid/1
  Serializer/1(serialOut) -> Interleaver/1(dataIn)
  Serializer/2(startOut) -> Interleaver/2(startIn)
  Serializer/3(endOut) -> Interleaver/3(endIn)
  Serializer/4(ValidOut) -> Interleaver/4(validIn)

== system gm_whdlOFDMTx/Frame Generator/Pilot ==
  note: Access pilot signals from LUT.
  pilot set : Inport  OutDataTypeStr=boolean  PortDimensions=1  SampleTime=4.8828125e-07
  Delay : Delay  DelayLength=1
  Delay2 : Delay  DelayLength=1
  Pilot Counter : hdlsllib/Sources/HDL Counter  CountType=Count limited  CountInit=0  CountStep=1  CountMax=length(pilotValPerSym) -1  CountFromType=Initial value  CountFrom=0  CountResetPort=off  CountLoadPort=off  CountEnbPort=on  CountDirPort=off  CountHitOutputPort=off  CountDataType=Unsigned  CountWordLen=nextpow2(length(pilotValPerSym) -1 +1)  CountFracLen=0  CountSampTime=1
  Pilot LUT : Lookup_n-D  NumberOfTableDimensions=1  LookupTableObject=''  BreakpointsForDimension1=0:(length(pilotValPerSym) -1)  BreakpointsForDimension1FirstPoint=10  BreakpointsForDimension2FirstPoint=10  BreakpointsForDimension1Spacing=12  BreakpointsForDimension2Spacing=12  IndexSearchMethod=Evenly spaced points  Table=pilotValPerSym  TableDataTypeStr=fixdt(1,16)  InterpMethod=Flat  DiagnosticForOutOfRangeInput=Error  InternalRulePriority=Speed  OutDataTypeStr=fixdt(1,16)  RndMeth=Simplest
  Upsample : dspsigops/Upsample  N=length(dataConvCode)  phase=0  RateOptions=Allow multirate processing  ic=0  mode=Unused parameter value
  Upsample1 : dspsigops/Upsample  N=length(dataConvCode)  phase=0  RateOptions=Allow multirate processing  ic=0  mode=Unused parameter value
  pilot : Outport  SampleTime=2.44140625e-07
  pilotValid : Outport  Port=2  SampleTime=2.44140625e-07
  wires:
  pilot set/1 -> Delay2/1, Pilot Counter/1
  Delay/1 -> Upsample/1
  Delay2/1 -> Upsample1/1
  Pilot Counter/1 -> Pilot LUT/1
  Pilot LUT/1 -> Delay/1
  Upsample/1 -> pilot/1
  Upsample1/1 -> pilotValid/1

== system gm_whdlOFDMTx/Frame Generator/Reference Signals ==
  note: Access reference signal from LUT.
  rs set : Inport  OutDataTypeStr=boolean  PortDimensions=1  SampleTime=4.8828125e-07
  Delay : Delay  DelayLength=1
  Delay2 : Delay  DelayLength=1
  RS Counter : hdlsllib/Sources/HDL Counter  CountType=Count limited  CountInit=0  CountStep=1  CountMax=length(rsSymbol) -1  CountFromType=Initial value  CountFrom=0  CountResetPort=off  CountLoadPort=off  CountEnbPort=on  CountDirPort=off  CountHitOutputPort=off  CountDataType=Unsigned  CountWordLen=nextpow2(length(rsSymbol) -1 +1)  CountFracLen=0  CountSampTime=1
  RS LUT : Lookup_n-D  NumberOfTableDimensions=1  LookupTableObject=''  BreakpointsForDimension1=0:(length(rsSymbol) -1)  BreakpointsForDimension1FirstPoint=10  BreakpointsForDimension2FirstPoint=10  BreakpointsForDimension1Spacing=12  BreakpointsForDimension2Spacing=12  IndexSearchMethod=Evenly spaced points  Table=rsSymbol  TableDataTypeStr=fixdt(1,16)  InterpMethod=Flat  DiagnosticForOutOfRangeInput=Error  InternalRulePriority=Speed  OutDataTypeStr=fixdt(1,16)  RndMeth=Simplest
  Upsample : dspsigops/Upsample  N=length(dataConvCode)  phase=0  RateOptions=Allow multirate processing  ic=0  mode=Unused parameter value
  Upsample1 : dspsigops/Upsample  N=length(dataConvCode)  phase=0  RateOptions=Allow multirate processing  ic=0  mode=Unused parameter value
  rs : Outport  SampleTime=2.44140625e-07
  rsValid : Outport  Port=2  SampleTime=2.44140625e-07
  wires:
  rs set/1 -> Delay2/1, RS Counter/1
  Delay/1 -> Upsample/1
  Delay2/1 -> Upsample1/1
  RS Counter/1 -> RS LUT/1
  RS LUT/1 -> Delay/1
  Upsample/1 -> rs/1
  Upsample1/1 -> rsValid/1

== system gm_whdlOFDMTx/Frame Generator/Synchronization Sequence ==
  note: Access synchronization sequence from LUT.
  ss set : Inport  OutDataTypeStr=boolean  PortDimensions=1  SampleTime=4.8828125e-07
  Delay : Delay  DelayLength=1
  Delay2 : Delay  DelayLength=1
  SS Counter : hdlsllib/Sources/HDL Counter  CountType=Count limited  CountInit=0  CountStep=1  CountMax=subC*NSS -1  CountFromType=Initial value  CountFrom=0  CountResetPort=off  CountLoadPort=off  CountEnbPort=on  CountDirPort=off  CountHitOutputPort=off  CountDataType=Unsigned  CountWordLen=nextpow2(subC*NSS -1 +1)  CountFracLen=0  CountSampTime=1
  SS LUT : Lookup_n-D  NumberOfTableDimensions=1  LookupTableObject=''  BreakpointsForDimension1=0:(length(ssSymbol)-1)  BreakpointsForDimension1FirstPoint=10  BreakpointsForDimension2FirstPoint=10  BreakpointsForDimension1Spacing=12  BreakpointsForDimension2Spacing=12  IndexSearchMethod=Evenly spaced points  Table=ssSymbol  TableDataTypeStr=fixdt(1,16)  InterpMethod=Flat  DiagnosticForOutOfRangeInput=Error  InternalRulePriority=Speed  OutDataTypeStr=fixdt(1,16)  RndMeth=Simplest
  Upsample : dspsigops/Upsample  N=length(dataConvCode)  phase=0  RateOptions=Allow multirate processing  ic=0  mode=Unused parameter value
  Upsample1 : dspsigops/Upsample  N=length(dataConvCode)  phase=0  RateOptions=Allow multirate processing  ic=0  mode=Unused parameter value
  ss : Outport  SampleTime=2.44140625e-07
  ssValid : Outport  Port=2  SampleTime=2.44140625e-07
  wires:
  ss set/1 -> Delay2/1, SS Counter/1
  Delay/1 -> Upsample/1
  Delay2/1 -> Upsample1/1
  SS Counter/1 -> SS LUT/1
  SS LUT/1 -> Delay/1
  Upsample/1 -> ss/1
  Upsample1/1 -> ssValid/1

== system gm_whdlOFDMTx/Multiplexer/Multiplex Header and Data Signals ==
  header : Inport  OutDataTypeStr=fixdt(1, 16, 14)  PortDimensions=1  SampleTime=2.44140625e-07
      settings: SignalType=complex
  headerValid : Inport  Port=2  OutDataTypeStr=boolean  PortDimensions=1  SampleTime=2.44140625e-07
  data : Inport  Port=3  OutDataTypeStr=fixdt(1, 16, 14)  PortDimensions=1  SampleTime=2.44140625e-07
      settings: SignalType=complex
  dataValid : Inport  Port=4  OutDataTypeStr=boolean  PortDimensions=1  SampleTime=2.44140625e-07
  Logical Operator : Logic  Operator=OR  IconShape=distinctive  AllPortsSameDT=off  OutDataTypeStr=boolean
  Switch : Switch  Criteria=u2 ~= 0  SaturateOnIntegerOverflow=off  InputSameDT=off
  dataOut : Outport  SampleTime=2.44140625e-07
  validOut : Outport  Port=2  SampleTime=2.44140625e-07
  wires:
  header/1 -> Switch/1
  headerValid/1 -> Switch/2, Logical Operator/1
  data/1 -> Switch/3
  dataValid/1 -> Logical Operator/2
  Logical Operator/1 -> validOut/1
  Switch/1 -> dataOut/1

== system gm_whdlOFDMTx/Multiplexer/Multiplex Preamble Signals ==
  ss : Inport  OutDataTypeStr=fixdt(1, 16, 14)  PortDimensions=1  SampleTime=2.44140625e-07
      settings: SignalType=complex
  ssValid : Inport  Port=2  OutDataTypeStr=boolean  PortDimensions=1  SampleTime=2.44140625e-07
  rs : Inport  Port=3  OutDataTypeStr=fixdt(1, 16, 14)  PortDimensions=1  SampleTime=2.44140625e-07
  rsValid : Inport  Port=4  OutDataTypeStr=boolean  PortDimensions=1  SampleTime=2.44140625e-07
  pilot : Inport  Port=5  OutDataTypeStr=fixdt(1, 16, 14)  PortDimensions=1  SampleTime=2.44140625e-07
  pilotValid : Inport  Port=6  OutDataTypeStr=boolean  PortDimensions=1  SampleTime=2.44140625e-07
  Logical Operator : Logic  Operator=OR  Inputs=3  IconShape=distinctive  AllPortsSameDT=off  OutDataTypeStr=boolean
  Multiport Switch : MultiPortSwitch  DataPortOrder=Zero-based contiguous  zeroidx=on  SaturateOnIntegerOverflow=off  InputSameDT=off
  Priority Encoder : Subsystem
  Real-Imag to Complex : RealImagToComplex  Input=Real
  Real-Imag to Complex1 : RealImagToComplex  Input=Real
  preambleOut : Outport  SampleTime=2.44140625e-07
  preambleValid : Outport  Port=2  SampleTime=2.44140625e-07
  wires:
  ss/1 -> Multiport Switch/2
  ssValid/1 -> Logical Operator/3, Priority Encoder/1(ssValid)
  rs/1 -> Real-Imag to Complex/1
  rsValid/1 -> Logical Operator/2, Priority Encoder/2(rsValid)
  pilot/1 -> Real-Imag to Complex1/1
  pilotValid/1 -> Logical Operator/1, Priority Encoder/3(pilotValid)
  Logical Operator/1 -> preambleValid/1
  Multiport Switch/1 -> preambleOut/1
  Priority Encoder/1(selLine) -> Multiport Switch/1
  Real-Imag to Complex/1 -> Multiport Switch/3
  Real-Imag to Complex1/1 -> Multiport Switch/4

== system gm_whdlOFDMTx/Frame Controller and Input Sampler/Enable Header and Preamble /Falling Edge Detector1 ==
  in : Inport  OutDataTypeStr=boolean  PortDimensions=1  SampleTime=4.8828125e-07
  Delay3 : Delay  DelayLength=1
  Logical Operator1 : Logic  IconShape=distinctive  AllPortsSameDT=off  OutDataTypeStr=boolean
  Logical Operator2 : Logic  Operator=NOT  IconShape=distinctive  AllPortsSameDT=off  OutDataTypeStr=boolean
  out : Outport  SampleTime=4.8828125e-07
  wires:
  in/1 -> Logical Operator2/1, Delay3/1
  Delay3/1 -> Logical Operator1/1
  Logical Operator1/1 -> out/1
  Logical Operator2/1 -> Logical Operator1/2

== system gm_whdlOFDMTx/Frame Controller and Input Sampler/Enable Header and Preamble /Falling Edge Detector2 ==
  in : Inport  OutDataTypeStr=boolean  PortDimensions=1  SampleTime=4.8828125e-07
  Delay3 : Delay  DelayLength=1
  Logical Operator1 : Logic  IconShape=distinctive  AllPortsSameDT=off  OutDataTypeStr=boolean
  Logical Operator2 : Logic  Operator=NOT  IconShape=distinctive  AllPortsSameDT=off  OutDataTypeStr=boolean
  out : Outport  SampleTime=4.8828125e-07
  wires:
  in/1 -> Logical Operator2/1, Delay3/1
  Delay3/1 -> Logical Operator1/1
  Logical Operator1/1 -> out/1
  Logical Operator2/1 -> Logical Operator1/2

== system gm_whdlOFDMTx/Frame Controller and Input Sampler/Enable Header and Preamble /MATLAB Function3 ==
  trigger : Inport  OutDataTypeStr=boolean  PortDimensions=1  SampleTime=4.8828125e-07
  MATLAB Function3 : MATLAB Function  TreatAsAtomicUnit=on  mask{nClocks=headerTime}
      mask prompts: nClocks "Number of clocks to hold:"
  out : Outport  SampleTime=4.8828125e-07  VectorParamsAs1DForOutWhenUnconnected=off
  wires:
  trigger/1 -> MATLAB Function3/1(trigger)
  MATLAB Function3/1(out) -> out/1

== system gm_whdlOFDMTx/Frame Controller and Input Sampler/Enable Header and Preamble /MATLAB Function4 ==
  trigger : Inport  OutDataTypeStr=boolean  PortDimensions=1  SampleTime=4.8828125e-07
  MATLAB Function4 : MATLAB Function  TreatAsAtomicUnit=on  mask{nClocks=NSS*subC + NRS*subC + pilotLen}
      mask prompts: nClocks "Number of clocks to hold:"
  out : Outport  SampleTime=4.8828125e-07  VectorParamsAs1DForOutWhenUnconnected=off
  wires:
  trigger/1 -> MATLAB Function4/1(trigger)
  MATLAB Function4/1(out) -> out/1

== system gm_whdlOFDMTx/Frame Controller and Input Sampler/Frame Controller/Generate OFDM Modulator Ready ==
  ready : Inport  OutDataTypeStr=boolean  PortDimensions=1  SampleTime=4.8828125e-07
  trBlkSize : Inport  Port=2  OutDataTypeStr=fixdt(0, 14, 0)  PortDimensions=1  SampleTime=4.8828125e-07
  Add : Sum  Inputs=+-  OutDataTypeStr=Inherit: Inherit via back propagation
  Compare To Constant1 : simulink/Logic and Bit Operations/Compare To Constant  relop===  const=(NSymPerF*(fftLen+cpLen))*rateFac2 - max(max(trBlkSize)) -4  OutDataTypeStr=boolean
  Constant : Constant  OutDataTypeStr=fixdt(0,1,0)  SampleTime=-1
  Control OFDM Signal Generation : Subsystem
  Delay1 : Delay  DelayLength=1
  HDL Counter1 : hdlsllib/Sources/HDL Counter  CountType=Count limited  CountInit=0  CountStep=1  CountMax=(NSymPerF*(fftLen+cpLen))*rateFac2  CountFromType=Initial value  CountFrom=0  CountResetPort=on  CountLoadPort=off  CountEnbPort=on  CountDirPort=off  CountHitOutputPort=off  CountDataType=Unsigned  CountWordLen="nextpow2((NSymPerF*(fftLen+cpLen))*rateFac2  +1)"  CountFracLen=0  CountSampTime=1
  Logical Operator : Logic  Operator=NOT  IconShape=distinctive  AllPortsSameDT=off  OutDataTypeStr=boolean
  Logical Operator5 : Logic  IconShape=distinctive  AllPortsSameDT=off  OutDataTypeStr=boolean
  Logical Operator7 : Logic  IconShape=distinctive  AllPortsSameDT=off  OutDataTypeStr=boolean
  MATLAB Function1 : Subsystem
  Relational Operator3 : RelationalOperator  Operator=<=  OutDataTypeStr=boolean  InputSameDT=off
  Rising Edge Detector : Subsystem
  resetRAM : Outport  SampleTime=4.8828125e-07
  dataSet : Outport  Port=2  SampleTime=4.8828125e-07
  ofdmModReady : Outport  Port=3  SampleTime=4.8828125e-07
  reset : Outport  Port=4  SampleTime=4.8828125e-07
  wires:
  ready/1 -> Logical Operator/1
  trBlkSize/1 -> Add/1
  Add/1 -> Relational Operator3/2
  Compare To Constant1/1 -> Delay1/1, reset/1
  Constant/1 -> Add/2
  Control OFDM Signal Generation/1(holdOFDMGen) -> Logical Operator7/2
  Delay1/1 -> Control OFDM Signal Generation/2(reset)
  HDL Counter1/1 -> Relational Operator3/1, Compare To Constant1/1
  Logical Operator/1 -> Logical Operator7/1, Control OFDM Signal Generation/1(readyLow)
  Logical Operator5/1 -> dataSet/1
  Logical Operator7/1 -> Rising Edge Detector/1(in)
  MATLAB Function1/1(out) -> Logical Operator5/1, ofdmModReady/1, HDL Counter1/2
  Relational Operator3/1 -> Logical Operator5/2
  Rising Edge Detector/1(out) -> MATLAB Function1/1(trigger), resetRAM/1, HDL Counter1/1
